simulink model "SVM"  (R2018b)
settings: Solver=VariableStepAuto  StartTime=0.0  StopTime=0.1  FixedStep=1/100000000  RelTol=1e-3
PostLoadFcn:
  | , if any(exist('dsrtsu_mdlpostloadfcn', 'file') ~= 0), dsrtsu_mdlpostloadfcn('Execute', bdroot); end,
values from neighbouring files (symbols this model uses):
  omega = 75    [param.m]
  Vo = 200    [param.m]
libraries: xbsIndex_r4 x2079, xrbsSSR_Library x20, xrbsMath_r4 x11, rtiproclib x6, rtifpgainterfacelib x1, powerlib_meascontrol x1
(part 4 of 23)

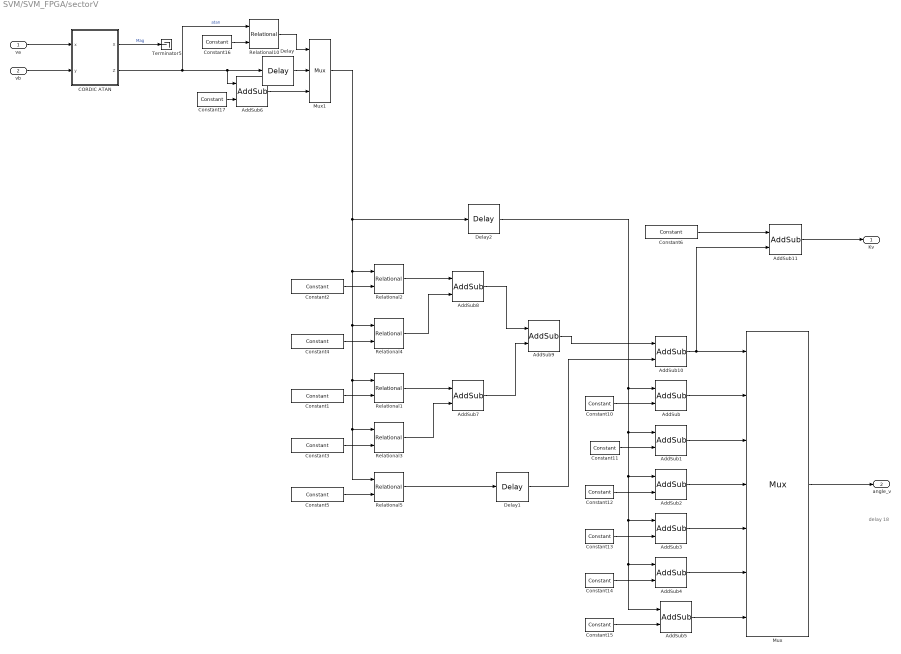
== system SVM/SVM_FPGA/sectorV ==
  note: delay 18
  va : Inport
  vb : Inport  Port=2
  AddSub{,1..5} (6 alike) : xbsIndex_r4/AddSub  mode=Subtraction  use_carryin=off  use_carryout=off  en=off  latency=1  precision=User Defined  arith_type="Signed  (2's comp)"  n_bits=16  bin_pt=8  quantization=Truncate  overflow=Wrap  use_behavioral_HDL=off  hw_selection=Fabric  pipelined=off  dbl_ovrd=off  block_type=addsub
  AddSub10 : xbsIndex_r4/AddSub  mode=Addition  use_carryin=off  use_carryout=off  en=off  latency=1  precision=User Defined  arith_type=Unsigned  n_bits=3  bin_pt=0  quantization=Truncate  overflow=Wrap  use_behavioral_HDL=off  hw_selection=Fabric  pipelined=off  dbl_ovrd=off  block_type=addsub
  AddSub11 : xbsIndex_r4/AddSub  mode=Addition  use_carryin=off  use_carryout=off  en=off  latency=1  precision=User Defined  arith_type=Unsigned  n_bits=3  bin_pt=0  quantization=Truncate  overflow=Wrap  use_behavioral_HDL=off  hw_selection=Fabric  pipelined=off  dbl_ovrd=off  block_type=addsub
  AddSub6 : xbsIndex_r4/AddSub  mode=Addition  use_carryin=off  use_carryout=off  en=off  latency=1  precision=User Defined  arith_type=Unsigned  n_bits=16  bin_pt=8  quantization=Truncate  overflow=Wrap  use_behavioral_HDL=off  hw_selection=Fabric  pipelined=off  dbl_ovrd=off  block_type=addsub
  AddSub7 : xbsIndex_r4/AddSub  mode=Addition  use_carryin=off  use_carryout=off  en=off  latency=1  precision=User Defined  arith_type=Unsigned  n_bits=2  bin_pt=0  quantization=Truncate  overflow=Wrap  use_behavioral_HDL=off  hw_selection=Fabric  pipelined=off  dbl_ovrd=off  block_type=addsub
  AddSub8 : xbsIndex_r4/AddSub  mode=Addition  use_carryin=off  use_carryout=off  en=off  latency=1  precision=User Defined  arith_type=Unsigned  n_bits=2  bin_pt=0  quantization=Truncate  overflow=Wrap  use_behavioral_HDL=off  hw_selection=Fabric  pipelined=off  dbl_ovrd=off  block_type=addsub
  AddSub9 : xbsIndex_r4/AddSub  mode=Addition  use_carryin=off  use_carryout=off  en=off  latency=1  precision=User Defined  arith_type=Unsigned  n_bits=3  bin_pt=0  quantization=Truncate  overflow=Wrap  use_behavioral_HDL=off  hw_selection=Fabric  pipelined=off  dbl_ovrd=off  block_type=addsub
  CORDIC ATAN : Subsystem  mask(Xilinx CORDIC ATAN){stages=25, pe_nbits=32, pe_binpt=8, pipeline_x=ones(1,8), prev_stages=25, pipeline=[1  1  1  1  1  1  1  1  0  0  0  0  0  0  0  0  0  0  0  0  0  0  0  0  0]}
      mask prompts: stages "Number of Processing Elements (integer value starting from 1)"; pe_nbits "X, Y Data Width"; pe_binpt "X, Y Binary Point Position"; pipeline_x "Latency for each Processing Element [1 0 0 1]"; prev_stages "Previous Number of Stages"; pipeline "Previous Pipeline Values"
      mask help: A parallel implementation, circular vectoring mode CORDIC processor for performing rectangular-to-polar conversion. The number of iteration stages (and resultant output accuracy) and the processor arithmetic precision are controlled by the mask customization.
      mask init:
      | [bg,fg] = xlcmap('XBlock',0);
      | iPos = get_param(gcb,'Position');
      | iWidth=iPos(3)-iPos(1); iHeight=iPos(4)-iPos(2);
      | iCx=iWidth/2;
      | iCy=iHeight/2;
      | [logoX, logoY] = xlogo(iPos);
      | sav_gcb=gcb;
      | stages = round(sum(abs(stages)));
      | if (stages == 0)
      | 	stages = prev_stages;
      | end
      | x = zeros(1,stages);
      | pipe_size = max(size(pipeline_x));
      | if pipe_size >= stages
      | 	x(1,1:stages) = pipeline_x(1,1:stages);
      | else
      | 	x(1,1:pipe_size) = pipeline_x(1,1:pipe_size);
      | end
      | 
      | if (stages ~=prev_stages)
      | 	pipeline=x;
      | 	cordic_pe = find_system(gcb, 'lookUnderMasks', 'all', 'FollowLinks','on','masktype', 'CORDIC parallel PE');
      |     
      |   a=find_system(cordic_pe{1}, 'lookUnderMasks', 'all', 'FollowLinks','on','masktype', 'CORDIC iteration PE');
      |   for i= 2:length(a)
      |     for j=1:3
      | 	  delete_line(cordic_pe{1}, ['CORDIC PE' int2str(i-1) '/' int2str(j)], ['CORDIC PE' int2str(i) '/' int2str(j)]);
      |     end
      |   end
      |     if length(a)>0,
      |       delete_line(cordic_pe{1}, 'x/1', 'CORDIC PE1/1');
      |       delete_line(cordic_pe{1}, 'y/1', 'CORDIC PE1/2');
      |       delete_line(cordic_pe{1}, 'z/1', 'CORDIC PE1/3');
      |       delete_line(cordic_pe{1}, ['CORDIC PE' int2str(length(a)) '/1'],'X/1');
      |       delete_line(cordic_pe{1}, ['CORDIC PE' int2str(length(a)) '/2'],'Terminator/1');
      |       delete_line(cordic_pe{1}, ['CORDIC PE' int2str(length(a)) '/3'],'Z/1');
      |     elseif length(a)==0
      |       temp_port=get_param([cordic_pe{1} '/x'],'porthandles');
      |       temp_line=get_param(temp_port.Outport,'line');
      |       if temp_line>=0  delete_line(temp_line); end
      |       temp_port=get_param([cordic_pe{1} '/y'],'porthandles');
      |       temp_line=get_param(temp_port.Outport,'line');
      |       if temp_line>=0  delete_line(temp_line); end
      |       temp_port=get_param([cordic_pe{1} '/z'],'porthandles');
      |       temp_line=get_param(temp_port.Outport,'line');
      |       if temp_line>=0  delete_line(temp_line); end
      |     end
      | 
      |     for i=2:length(a)
      |       delete_block(a{i});
      |     end
      |     for i=2:stages,
      |         add_block([cordic_pe{1} '/CORDIC PE1'], [cordic_pe{1} '/CORDIC PE' int2str(i)], 'ii', int2str(i-1),'pe_nbits', 'pe_nbits','pe_binpt', 'pe_binpt','pipeline',['pipeline(1,' int2str(i) ')'],'position',[150+(i-1)*125, 70, 205+(i-1)*125, 130]);
      |     end
      | 
      |     for i= 2:stages,
      |       for j=1:3
      | 		add_line(cordic_pe{1}, ['CORDIC PE' int2str(i-1) '/' int2str(j)], ['CORDIC PE' int2str(i) '/' int2str(j)], 'autorouting', 'on');
      |       end
      |     end
      | 
      |     if stages==0
      |       add_line(cordic_pe{1}, 'x/1', 'X/1', 'autorouting', 'on');
      |       add_line(cordic_pe{1}, 'y/1', 'Terminator/1', 'autorouting', 'on');
      |       add_line(cordic_pe{1}, 'z/1', 'Z/1', 'autorouting', 'on');
      |     elseif stages>0
      |       add_line(cordic_pe{1}, 'x/1', 'CORDIC PE1/1', 'autorouting', 'on');
      |       add_line(cordic_pe{1}, 'y/1', 'CORDIC PE1/2', 'autorouting', 'on');
      |       add_line(cordic_pe{1}, 'z/1', 'CORDIC PE1/3', 'autorouting', 'on');
      | 
      |       set_param([cordic_pe{1} '/' 'X'], 'Position', [150+stages*125, 72, 180+stages*125, 86]);
      |       set_param([cordic_pe{1} '/' 'Terminator'], 'Position', [210+stages*125, 92, 225+stages*125, 108]);
      |       set_param([cordic_pe{1} '/' 'Z'], 'Position', [240+stages*125, 113, 270+stages*125, 127]);
      | 
      |       add_line(cordic_pe{1}, ['CORDIC PE' int2str(stages) '/1'], 'X/1', 'autorouting', 'on');
      |       add_line(cordic_pe{1}, ['CORDIC PE' int2str(stages) '/2'], 'Terminator/1', 'autorouting', 'on');
      |       add_line(cordic_pe{1}, ['CORDIC PE' int2str(stages) '/3'],'Z/1', 'autorouting', 'on');
      | 
      |       % force a "compile" of the constituent constant blocks to
      |       % workaround a data propagation problem
      |       find_system(cordic_pe{1}, 'lookUnderMasks', 'all', 'FollowLinks', 'on', 'MaskType','Xilinx Constant Block');
      |   end
      | 	set_param(sav_gcb, 'prev_stages', int2str(stages));
      | 	set_param(sav_gcb, 'pipeline', [ '[' int2str(x) ']']);
      | else
      | 	if (sum(pipeline~=x))
      | 		set_param(gcb, 'pipeline', [ '[' int2str(x) ']']);
      | 	end
      | end
      | str = sprintf('-%d',sum(x) + 3);
      settings: CopyFcn=set_param(gcb, 'MaskSelfModifiable', 'on', 'LinkStatus', 'none');
      mask Help: eval('');xlDoc('-book','sysgen','-topic','CORDIC_ATAN');
      mask Display:
      | patch([0 iWidth iWidth 0],[0 0 iHeight iHeight] , bg);
      | patch(logoX,logoY , fg);
      | text(iCx-6,iCy,'z');
      | text(iCx,iCy+4,str);
      | port_label('input',1,'x');
      | port_label('input',2,'y');
      | port_label('output',1,'mag');
      | port_label('output',2,'atan');
      | plot([0 0 iWidth iWidth 0], [0 iHeight iHeight 0 0]);
  Constant1 : xbsIndex_r4/Constant  const=pi  gui_display_data_type=Fixed-point  arith_type=Signed (2's comp)  n_bits=16  bin_pt=8  preci_type=Single  exp_width=8  frac_width=24  explicit_period=off  period=1  equ=P=C  opselect=C  inp2=PCIN>>17  opr=+  inp1=P  carry=CIN  dbl_ovrd=off  block_type=constant
  Constant10 : xbsIndex_r4/Constant  const=pi/6  gui_display_data_type=Fixed-point  arith_type=Signed (2's comp)  n_bits=16  bin_pt=8  preci_type=Single  exp_width=8  frac_width=24  explicit_period=off  period=1  equ=P=C  opselect=C  inp2=PCIN>>17  opr=+  inp1=P  carry=CIN  dbl_ovrd=off  block_type=constant
  Constant11 : xbsIndex_r4/Constant  const=pi/2  gui_display_data_type=Fixed-point  arith_type=Signed (2's comp)  n_bits=16  bin_pt=8  preci_type=Single  exp_width=8  frac_width=24  explicit_period=off  period=1  equ=P=C  opselect=C  inp2=PCIN>>17  opr=+  inp1=P  carry=CIN  dbl_ovrd=off  block_type=constant
  Constant12 : xbsIndex_r4/Constant  const=5*pi/6  gui_display_data_type=Fixed-point  arith_type=Signed (2's comp)  n_bits=16  bin_pt=8  preci_type=Single  exp_width=8  frac_width=24  explicit_period=off  period=1  equ=P=C  opselect=C  inp2=PCIN>>17  opr=+  inp1=P  carry=CIN  dbl_ovrd=off  block_type=constant
  Constant13 : xbsIndex_r4/Constant  const=7*pi/6  gui_display_data_type=Fixed-point  arith_type=Signed (2's comp)  n_bits=16  bin_pt=8  preci_type=Single  exp_width=8  frac_width=24  explicit_period=off  period=1  equ=P=C  opselect=C  inp2=PCIN>>17  opr=+  inp1=P  carry=CIN  dbl_ovrd=off  block_type=constant
  Constant14 : xbsIndex_r4/Constant  const=3*pi/2  gui_display_data_type=Fixed-point  arith_type=Signed (2's comp)  n_bits=16  bin_pt=8  preci_type=Single  exp_width=8  frac_width=24  explicit_period=off  period=1  equ=P=C  opselect=C  inp2=PCIN>>17  opr=+  inp1=P  carry=CIN  dbl_ovrd=off  block_type=constant
  Constant15 : xbsIndex_r4/Constant  const=11*pi/6  gui_display_data_type=Fixed-point  arith_type=Signed (2's comp)  n_bits=16  bin_pt=8  preci_type=Single  exp_width=8  frac_width=24  explicit_period=off  period=1  equ=P=C  opselect=C  inp2=PCIN>>17  opr=+  inp1=P  carry=CIN  dbl_ovrd=off  block_type=constant
  Constant16 : xbsIndex_r4/Constant  const=0.0  gui_display_data_type=Fixed-point  arith_type=Signed (2's comp)  n_bits=16  bin_pt=8  preci_type=Single  exp_width=8  frac_width=24  explicit_period=off  period=1  equ=P=C  opselect=C  inp2=PCIN>>17  opr=+  inp1=P  carry=CIN  dbl_ovrd=off  block_type=constant
  Constant17 : xbsIndex_r4/Constant  const=2*pi  gui_display_data_type=Fixed-point  arith_type=Signed (2's comp)  n_bits=16  bin_pt=8  preci_type=Single  exp_width=8  frac_width=24  explicit_period=off  period=1  equ=P=C  opselect=C  inp2=PCIN>>17  opr=+  inp1=P  carry=CIN  dbl_ovrd=off  block_type=constant
  Constant2 : xbsIndex_r4/Constant  const=pi/3  gui_display_data_type=Fixed-point  arith_type=Signed (2's comp)  n_bits=16  bin_pt=8  preci_type=Single  exp_width=8  frac_width=24  explicit_period=off  period=1  equ=P=C  opselect=C  inp2=PCIN>>17  opr=+  inp1=P  carry=CIN  dbl_ovrd=off  block_type=constant
  Constant3 : xbsIndex_r4/Constant  const=4*pi/3  gui_display_data_type=Fixed-point  arith_type=Signed (2's comp)  n_bits=16  bin_pt=8  preci_type=Single  exp_width=8  frac_width=24  explicit_period=off  period=1  equ=P=C  opselect=C  inp2=PCIN>>17  opr=+  inp1=P  carry=CIN  dbl_ovrd=off  block_type=constant
  Constant4 : xbsIndex_r4/Constant  const=2*pi/3  gui_display_data_type=Fixed-point  arith_type=Signed (2's comp)  n_bits=16  bin_pt=8  preci_type=Single  exp_width=8  frac_width=24  explicit_period=off  period=1  equ=P=C  opselect=C  inp2=PCIN>>17  opr=+  inp1=P  carry=CIN  dbl_ovrd=off  block_type=constant
  Constant5 : xbsIndex_r4/Constant  const=5*pi/3  gui_display_data_type=Fixed-point  arith_type=Signed (2's comp)  n_bits=16  bin_pt=8  preci_type=Single  exp_width=8  frac_width=24  explicit_period=off  period=1  equ=P=C  opselect=C  inp2=PCIN>>17  opr=+  inp1=P  carry=CIN  dbl_ovrd=off  block_type=constant
  Constant6 : xbsIndex_r4/Constant  const=1  gui_display_data_type=Fixed-point  arith_type=Signed (2's comp)  n_bits=3  bin_pt=0  preci_type=Single  exp_width=8  frac_width=24  explicit_period=off  period=1  equ=P=C  opselect=C  inp2=PCIN>>17  opr=+  inp1=P  carry=CIN  dbl_ovrd=off  block_type=constant
  Delay : xbsIndex_r4/Delay  rst=off  infoeditControl=Selection of Reset will increase slice count due to use of real FFs and instead of SRLs  en=off  latency=1  reg_retiming=off  dbl_ovrd=off  block_type=delay
  Delay1 : xbsIndex_r4/Delay  rst=off  infoeditControl=Selection of Reset will increase slice count due to use of real FFs and instead of SRLs  en=off  latency=2  reg_retiming=off  dbl_ovrd=off  block_type=delay
  Delay2 : xbsIndex_r4/Delay  rst=off  infoeditControl=Selection of Reset will increase slice count due to use of real FFs and instead of SRLs  en=off  latency=3  reg_retiming=off  dbl_ovrd=off  block_type=delay
  Mux : xbsIndex_r4/Mux  inputs=6  en=off  latency=1  precision=User Defined  arith_type="Signed  (2's comp)"  n_bits=16  bin_pt=8  quantization=Truncate  overflow=Wrap  dbl_ovrd=off  block_type=mux
  Mux1 : xbsIndex_r4/Mux  inputs=2  en=off  latency=1  precision=User Defined  arith_type="Signed  (2's comp)"  n_bits=16  bin_pt=8  quantization=Truncate  overflow=Wrap  dbl_ovrd=off  block_type=mux
  Relational{1..5} (5 alike) : xbsIndex_r4/Relational  mode=a>=b  op_type=Ufix  en=off  latency=1  dbl_ovrd=off  block_type=relational
  Relational10 : xbsIndex_r4/Relational  mode=a<b  op_type=Bool  en=off  latency=1  dbl_ovrd=off  block_type=relational
  Terminator5 : Terminator
  Kv : Outport
  angle_v : Outport  Port=2
  wires:
  Constant14/1 -> AddSub4/2
  Constant12/1 -> AddSub2/2
  Constant10/1 -> AddSub/2
  Delay1/1 -> AddSub10/2
  Constant11/1 -> AddSub1/2
  Relational2/1 -> AddSub8/1
  Constant5/1 -> Relational5/2
  Delay2/1 -> AddSub4/1, AddSub5/1, AddSub3/1, AddSub2/1, AddSub1/1, AddSub/1
  va/1 -> CORDIC ATAN/1(x)
  Constant4/1 -> Relational4/2
  Mux1/1 -> Relational5/1, Relational3/1, Relational1/1, Relational4/1, Relational2/1, Delay2/1
  Constant16/1 -> Relational10/2
  CORDIC ATAN/1(X) -> Terminator5/1  "Mag"
  Constant17/1 -> AddSub6/2
  AddSub/1 -> Mux/2
  AddSub2/1 -> Mux/4
  AddSub5/1 -> Mux/7
  CORDIC ATAN/2(Z) -> Relational10/1, AddSub6/1, Delay/1  "atan"
  vb/1 -> CORDIC ATAN/2(y)
  Delay/1 -> Mux1/2
  Relational4/1 -> AddSub8/2
  Constant2/1 -> Relational2/2
  AddSub8/1 -> AddSub9/1
  AddSub1/1 -> Mux/3
  Relational1/1 -> AddSub7/1
  Constant3/1 -> Relational3/2
  Relational10/1 -> Mux1/1
  AddSub9/1 -> AddSub10/1
  AddSub11/1 -> Kv/1
  Constant1/1 -> Relational1/2
  AddSub4/1 -> Mux/6
  Relational3/1 -> AddSub7/2
  AddSub6/1 -> Mux1/3
  AddSub3/1 -> Mux/5
  AddSub7/1 -> AddSub9/2
  Constant6/1 -> AddSub11/1
  Relational5/1 -> Delay1/1
  Constant13/1 -> AddSub3/2
  AddSub10/1 -> AddSub11/2, Mux/1
  Constant15/1 -> AddSub5/2
  Mux/1 -> angle_v/1

== system SVM/SVM_FPGA/select_vector ==
  vector : Inport
  +1 : xbsIndex_r4/Constant  const=19  gui_display_data_type=Fixed-point  arith_type=Unsigned  n_bits=9  bin_pt=0  preci_type=Single  exp_width=8  frac_width=24  explicit_period=off  period=1  equ=P=C  opselect=C  inp2=PCIN>>17  opr=+  inp1=P  carry=CIN  dbl_ovrd=off  block_type=constant
  +{2..9} (8 alike) : xbsIndex_r4/Constant  const=19  gui_display_data_type=Fixed-point  arith_type=Signed (2's comp)  n_bits=16  bin_pt=8  preci_type=Single  exp_width=8  frac_width=24  explicit_period=off  period=1  equ=P=C  opselect=C  inp2=PCIN>>17  opr=+  inp1=P  carry=CIN  dbl_ovrd=off  block_type=constant
  -{1..9} (9 alike) : xbsIndex_r4/Constant  const=19  gui_display_data_type=Fixed-point  arith_type=Signed (2's comp)  n_bits=16  bin_pt=8  preci_type=Single  exp_width=8  frac_width=24  explicit_period=off  period=1  equ=P=C  opselect=C  inp2=PCIN>>17  opr=+  inp1=P  carry=CIN  dbl_ovrd=off  block_type=constant
  0a : xbsIndex_r4/Constant  const=19  gui_display_data_type=Fixed-point  arith_type=Signed (2's comp)  n_bits=16  bin_pt=8  preci_type=Single  exp_width=8  frac_width=24  explicit_period=off  period=1  equ=P=C  opselect=C  inp2=PCIN>>17  opr=+  inp1=P  carry=CIN  dbl_ovrd=off  block_type=constant
  0b : xbsIndex_r4/Constant  const=19  gui_display_data_type=Fixed-point  arith_type=Signed (2's comp)  n_bits=16  bin_pt=8  preci_type=Single  exp_width=8  frac_width=24  explicit_period=off  period=1  equ=P=C  opselect=C  inp2=PCIN>>17  opr=+  inp1=P  carry=CIN  dbl_ovrd=off  block_type=constant
  0c : xbsIndex_r4/Constant  const=19  gui_display_data_type=Fixed-point  arith_type=Signed (2's comp)  n_bits=16  bin_pt=8  preci_type=Single  exp_width=8  frac_width=24  explicit_period=off  period=1  equ=P=C  opselect=C  inp2=PCIN>>17  opr=+  inp1=P  carry=CIN  dbl_ovrd=off  block_type=constant
  Mux1 : xbsIndex_r4/Mux  inputs=21  en=off  latency=1  precision=Full  arith_type=Unsigned  n_bits=16  bin_pt=14  quantization=Truncate  overflow=Wrap  dbl_ovrd=off  block_type=mux
  switches : Outport
  wires:
  +3/1 -> Mux1/6
  +2/1 -> Mux1/4
  +1/1 -> Mux1/2
  +7/1 -> Mux1/14
  +8/1 -> Mux1/16
  -2/1 -> Mux1/5
  -3/1 -> Mux1/7
  -4/1 -> Mux1/9
  -7/1 -> Mux1/15
  +5/1 -> Mux1/10
  0c/1 -> Mux1/22
  0b/1 -> Mux1/21
  -8/1 -> Mux1/17
  +4/1 -> Mux1/8
  +9/1 -> Mux1/18
  +6/1 -> Mux1/12
  -5/1 -> Mux1/11
  vector/1 -> Mux1/1
  -6/1 -> Mux1/13
  -9/1 -> Mux1/19
  -1/1 -> Mux1/3
  0a/1 -> Mux1/20
  Mux1/1 -> switches/1

== system SVM/SVM_FPGA/ticks_calculator ==
  note: delay 6
  ticks_per_period : Inport
  d1 : Inport  Port=2
  d2 : Inport  Port=3
  d3 : Inport  Port=4
  d4 : Inport  Port=5
  AddSub : xbsIndex_r4/AddSub  mode=Addition  use_carryin=off  use_carryout=off  en=off  latency=1  precision=Full  arith_type=Unsigned  n_bits=16  bin_pt=14  quantization=Truncate  overflow=Wrap  use_behavioral_HDL=off  hw_selection=Fabric  pipelined=off  dbl_ovrd=off  block_type=addsub
  AddSub1 : xbsIndex_r4/AddSub  mode=Addition  use_carryin=off  use_carryout=off  en=off  latency=1  precision=Full  arith_type=Unsigned  n_bits=16  bin_pt=14  quantization=Truncate  overflow=Wrap  use_behavioral_HDL=off  hw_selection=Fabric  pipelined=off  dbl_ovrd=off  block_type=addsub
  AddSub2 : xbsIndex_r4/AddSub  mode=Subtraction  use_carryin=off  use_carryout=off  en=off  latency=1  precision=Full  arith_type=Unsigned  n_bits=16  bin_pt=14  quantization=Truncate  overflow=Wrap  use_behavioral_HDL=off  hw_selection=Fabric  pipelined=off  dbl_ovrd=off  block_type=addsub
  AddSub3 : xbsIndex_r4/AddSub  mode=Addition  use_carryin=off  use_carryout=off  en=off  latency=1  precision=Full  arith_type=Unsigned  n_bits=16  bin_pt=14  quantization=Truncate  overflow=Wrap  use_behavioral_HDL=off  hw_selection=Fabric  pipelined=off  dbl_ovrd=off  block_type=addsub
  Delay{,1..3} (4 alike) : xbsIndex_r4/Delay  rst=off  infoeditControl=Selection of Reset will increase slice count due to use of real FFs and instead of SRLs  en=off  latency=3  reg_retiming=off  dbl_ovrd=off  block_type=delay
  Mult{,1..3} (4 alike) : xbsIndex_r4/Mult  precision=Full  arith_type="Signed  (2's comp)"  n_bits=16  bin_pt=14  quantization=Truncate  overflow=Wrap  en=off  latency=3  use_behavioral_HDL=off  opt=Speed  use_embedded=on  optimum_pipeline=off  pipeline=on  dbl_ovrd=off  use_rpm=on  placement_style=Triangular  block_type=mult
  d0_counts : Outport
  d1_counts : Outport  Port=2
  d2_counts : Outport  Port=3
  d3_counts : Outport  Port=4
  "d4_counts " : Outport  Port=5
  wires:
  ticks_per_period/1 -> AddSub2/1, Mult1/2, Mult2/2, Mult3/2, Mult/2
  Mult/1 -> Delay/1, AddSub/1
  d1/1 -> Mult/1
  Mult2/1 -> AddSub1/1, Delay2/1
  d4/1 -> Mult3/1
  Mult3/1 -> Delay3/1, AddSub1/2
  AddSub1/1 -> AddSub3/2
  Mult1/1 -> Delay1/1, AddSub/2
  d2/1 -> Mult1/1
  AddSub/1 -> AddSub3/1
  AddSub3/1 -> AddSub2/2
  d3/1 -> Mult2/1
  AddSub2/1 -> d0_counts/1
  Delay/1 -> d1_counts/1
  Delay1/1 -> d2_counts/1
  Delay2/1 -> d3_counts/1
  Delay3/1 -> "d4_counts "/1

== system SVM/SVM_FPGA/vector_selector ==
  note: delay 1
  sector : Inport
  Demux : Demux
  Vector Constant : xrbsSSR_Library/Vector Constant  const=[17 14 6 1]  gui_display_data_type=Fixed-point  arith_type=Signed (2's comp)  n_bits=5  bin_pt=0  preci_type=Single  exp_width=8  frac_width=24  explicit_period=off  period=1  sg_ssr=4  sg_ssr_prev=4  equ=P=C  opselect=C  inp2=PCIN>>17  opr=+  inp1=P  carry=CIN  dbl_ovrd=off  block_type=constant_ssr
      settings: SourceProductName=Xilinx SSR Blockset
  Vector Constant1 : xrbsSSR_Library/Vector Constant  const=[16 17 3 6]  gui_display_data_type=Fixed-point  arith_type=Signed (2's comp)  n_bits=5  bin_pt=0  preci_type=Single  exp_width=8  frac_width=24  explicit_period=off  period=1  sg_ssr=4  sg_ssr_prev=4  equ=P=C  opselect=C  inp2=PCIN>>17  opr=+  inp1=P  carry=CIN  dbl_ovrd=off  block_type=constant_ssr
      settings: SourceProductName=Xilinx SSR Blockset
  Vector Constant10 : xrbsSSR_Library/Vector Constant  const=[15 18 4 5]  gui_display_data_type=Fixed-point  arith_type=Signed (2's comp)  n_bits=5  bin_pt=0  preci_type=Single  exp_width=8  frac_width=24  explicit_period=off  period=1  sg_ssr=4  sg_ssr_prev=4  equ=P=C  opselect=C  inp2=PCIN>>17  opr=+  inp1=P  carry=CIN  dbl_ovrd=off  block_type=constant_ssr
      settings: SourceProductName=Xilinx SSR Blockset
  Vector Constant11 : xrbsSSR_Library/Vector Constant  const=[14 15 1 4]  gui_display_data_type=Fixed-point  arith_type=Signed (2's comp)  n_bits=5  bin_pt=0  preci_type=Single  exp_width=8  frac_width=24  explicit_period=off  period=1  sg_ssr=4  sg_ssr_prev=4  equ=P=C  opselect=C  inp2=PCIN>>17  opr=+  inp1=P  carry=CIN  dbl_ovrd=off  block_type=constant_ssr
      settings: SourceProductName=Xilinx SSR Blockset
  Vector Constant12 : xrbsSSR_Library/Vector Constant  const=[11 8 18 13]  gui_display_data_type=Fixed-point  arith_type=Signed (2's comp)  n_bits=5  bin_pt=0  preci_type=Single  exp_width=8  frac_width=24  explicit_period=off  period=1  sg_ssr=4  sg_ssr_prev=4  equ=P=C  opselect=C  inp2=PCIN>>17  opr=+  inp1=P  carry=CIN  dbl_ovrd=off  block_type=constant_ssr
      settings: SourceProductName=Xilinx SSR Blockset
  Vector Constant13 : xrbsSSR_Library/Vector Constant  const=[10 11 15 18]  gui_display_data_type=Fixed-point  arith_type=Signed (2's comp)  n_bits=5  bin_pt=0  preci_type=Single  exp_width=8  frac_width=24  explicit_period=off  period=1  sg_ssr=4  sg_ssr_prev=4  equ=P=C  opselect=C  inp2=PCIN>>17  opr=+  inp1=P  carry=CIN  dbl_ovrd=off  block_type=constant_ssr
      settings: SourceProductName=Xilinx SSR Blockset
  Vector Constant14 : xrbsSSR_Library/Vector Constant  const=[7 10 14 15]  gui_display_data_type=Fixed-point  arith_type=Signed (2's comp)  n_bits=5  bin_pt=0  preci_type=Single  exp_width=8  frac_width=24  explicit_period=off  period=1  sg_ssr=4  sg_ssr_prev=4  equ=P=C  opselect=C  inp2=PCIN>>17  opr=+  inp1=P  carry=CIN  dbl_ovrd=off  block_type=constant_ssr
      settings: SourceProductName=Xilinx SSR Blockset
  Vector Constant15 : xrbsSSR_Library/Vector Constant  const=[6 1 11 8]  gui_display_data_type=Fixed-point  arith_type=Signed (2's comp)  n_bits=5  bin_pt=0  preci_type=Single  exp_width=8  frac_width=24  explicit_period=off  period=1  sg_ssr=4  sg_ssr_prev=4  equ=P=C  opselect=C  inp2=PCIN>>17  opr=+  inp1=P  carry=CIN  dbl_ovrd=off  block_type=constant_ssr
      settings: SourceProductName=Xilinx SSR Blockset
  Vector Constant16 : xrbsSSR_Library/Vector Constant  const=[3 6 10 11]  gui_display_data_type=Fixed-point  arith_type=Signed (2's comp)  n_bits=5  bin_pt=0  preci_type=Single  exp_width=8  frac_width=24  explicit_period=off  period=1  sg_ssr=4  sg_ssr_prev=4  equ=P=C  opselect=C  inp2=PCIN>>17  opr=+  inp1=P  carry=CIN  dbl_ovrd=off  block_type=constant_ssr
      settings: SourceProductName=Xilinx SSR Blockset
  Vector Constant17 : xrbsSSR_Library/Vector Constant  const=[2 3 7 10]  gui_display_data_type=Fixed-point  arith_type=Signed (2's comp)  n_bits=5  bin_pt=0  preci_type=Single  exp_width=8  frac_width=24  explicit_period=off  period=1  sg_ssr=4  sg_ssr_prev=4  equ=P=C  opselect=C  inp2=PCIN>>17  opr=+  inp1=P  carry=CIN  dbl_ovrd=off  block_type=constant_ssr
      settings: SourceProductName=Xilinx SSR Blockset
  Vector Constant18 : xrbsSSR_Library/Vector Constant  const=[19 19 19 19]  gui_display_data_type=Fixed-point  arith_type=Signed (2's comp)  n_bits=5  bin_pt=0  preci_type=Single  exp_width=8  frac_width=24  explicit_period=off  period=1  sg_ssr=4  sg_ssr_prev=4  equ=P=C  opselect=C  inp2=PCIN>>17  opr=+  inp1=P  carry=CIN  dbl_ovrd=off  block_type=constant_ssr
      settings: SourceProductName=Xilinx SSR Blockset
  Vector Constant2 : xrbsSSR_Library/Vector Constant  const=[13 16 2 3]  gui_display_data_type=Fixed-point  arith_type=Signed (2's comp)  n_bits=5  bin_pt=0  preci_type=Single  exp_width=8  frac_width=24  explicit_period=off  period=1  sg_ssr=4  sg_ssr_prev=4  equ=P=C  opselect=C  inp2=PCIN>>17  opr=+  inp1=P  carry=CIN  dbl_ovrd=off  block_type=constant_ssr
      settings: SourceProductName=Xilinx SSR Blockset
  Vector Constant3 : xrbsSSR_Library/Vector Constant  const=[12 7 17 14]  gui_display_data_type=Fixed-point  arith_type=Signed (2's comp)  n_bits=5  bin_pt=0  preci_type=Single  exp_width=8  frac_width=24  explicit_period=off  period=1  sg_ssr=4  sg_ssr_prev=4  equ=P=C  opselect=C  inp2=PCIN>>17  opr=+  inp1=P  carry=CIN  dbl_ovrd=off  block_type=constant_ssr
      settings: SourceProductName=Xilinx SSR Blockset
  Vector Constant4 : xrbsSSR_Library/Vector Constant  const=[9 12 16 17]  gui_display_data_type=Fixed-point  arith_type=Signed (2's comp)  n_bits=5  bin_pt=0  preci_type=Single  exp_width=8  frac_width=24  explicit_period=off  period=1  sg_ssr=4  sg_ssr_prev=4  equ=P=C  opselect=C  inp2=PCIN>>17  opr=+  inp1=P  carry=CIN  dbl_ovrd=off  block_type=constant_ssr
      settings: SourceProductName=Xilinx SSR Blockset
  Vector Constant5 : xrbsSSR_Library/Vector Constant  const=[8 9 13 16]  gui_display_data_type=Fixed-point  arith_type=Signed (2's comp)  n_bits=5  bin_pt=0  preci_type=Single  exp_width=8  frac_width=24  explicit_period=off  period=1  sg_ssr=4  sg_ssr_prev=4  equ=P=C  opselect=C  inp2=PCIN>>17  opr=+  inp1=P  carry=CIN  dbl_ovrd=off  block_type=constant_ssr
      settings: SourceProductName=Xilinx SSR Blockset
  Vector Constant6 : xrbsSSR_Library/Vector Constant  const=[5 2 12 7]  gui_display_data_type=Fixed-point  arith_type=Signed (2's comp)  n_bits=5  bin_pt=0  preci_type=Single  exp_width=8  frac_width=24  explicit_period=off  period=1  sg_ssr=4  sg_ssr_prev=4  equ=P=C  opselect=C  inp2=PCIN>>17  opr=+  inp1=P  carry=CIN  dbl_ovrd=off  block_type=constant_ssr
      settings: SourceProductName=Xilinx SSR Blockset
  Vector Constant7 : xrbsSSR_Library/Vector Constant  const=[4 5 9 12]  gui_display_data_type=Fixed-point  arith_type=Signed (2's comp)  n_bits=5  bin_pt=0  preci_type=Single  exp_width=8  frac_width=24  explicit_period=off  period=1  sg_ssr=4  sg_ssr_prev=4  equ=P=C  opselect=C  inp2=PCIN>>17  opr=+  inp1=P  carry=CIN  dbl_ovrd=off  block_type=constant_ssr
      settings: SourceProductName=Xilinx SSR Blockset
  Vector Constant8 : xrbsSSR_Library/Vector Constant  const=[1 4 8 9]  gui_display_data_type=Fixed-point  arith_type=Signed (2's comp)  n_bits=5  bin_pt=0  preci_type=Single  exp_width=8  frac_width=24  explicit_period=off  period=1  sg_ssr=4  sg_ssr_prev=4  equ=P=C  opselect=C  inp2=PCIN>>17  opr=+  inp1=P  carry=CIN  dbl_ovrd=off  block_type=constant_ssr
      settings: SourceProductName=Xilinx SSR Blockset
  Vector Constant9 : xrbsSSR_Library/Vector Constant  const=[18 13 5 2]  gui_display_data_type=Fixed-point  arith_type=Signed (2's comp)  n_bits=5  bin_pt=0  preci_type=Single  exp_width=8  frac_width=24  explicit_period=off  period=1  sg_ssr=4  sg_ssr_prev=4  equ=P=C  opselect=C  inp2=PCIN>>17  opr=+  inp1=P  carry=CIN  dbl_ovrd=off  block_type=constant_ssr
      settings: SourceProductName=Xilinx SSR Blockset
  Vector Mux : xrbsSSR_Library/Vector Mux  inputs=32  inputs_prev=31  en=off  vectorize_en=off  vectorize_sel=off  sg_latency=1  precision=User Defined  arith_type=Unsigned  n_bits=16  bin_pt=0  quantization=Truncate  overflow=Wrap  dbl_ovrd=off  block_type=mux_ssr  sg_ssr=4  sg_ssr_prev=4  sg_ssr_name=vect_mux
      settings: SourceProductName=Xilinx SSR Blockset  infoedit=The Vector Multiplexer block supports Multiplexing feature for input of vector types.
  "v1 " : Outport
  v2 : Outport  Port=2
  v3 : Outport  Port=3
  "v4 " : Outport  Port=4
  wires:
  Vector Mux/1 -> Demux/1
  Vector Constant/1 -> Vector Mux/2
  Vector Constant1/1 -> Vector Mux/3
  Vector Constant3/1 -> Vector Mux/5
  sector/1 -> Vector Mux/1
  Demux/1 -> "v1 "/1
  Demux/2 -> v2/1
  Demux/3 -> v3/1
  Demux/4 -> "v4 "/1
  Vector Constant2/1 -> Vector Mux/4
  Vector Constant4/1 -> Vector Mux/6
  Vector Constant5/1 -> Vector Mux/7
  Vector Constant6/1 -> Vector Mux/8
  Vector Constant7/1 -> Vector Mux/9
  Vector Constant8/1 -> Vector Mux/10
  Vector Constant9/1 -> Vector Mux/11
  Vector Constant10/1 -> Vector Mux/12
  Vector Constant11/1 -> Vector Mux/13
  Vector Constant12/1 -> Vector Mux/14
  Vector Constant13/1 -> Vector Mux/15
  Vector Constant14/1 -> Vector Mux/16
  Vector Constant15/1 -> Vector Mux/17
  Vector Constant16/1 -> Vector Mux/18
  Vector Constant17/1 -> Vector Mux/19
  Vector Constant18/1 -> Vector Mux/20, Vector Mux/21, Vector Mux/22, Vector Mux/23, Vector Mux/24, Vector Mux/25, Vector Mux/26, Vector Mux/27, Vector Mux/28, Vector Mux/29, Vector Mux/30, Vector Mux/31, Vector Mux/32, Vector Mux/33

== system SVM/SVM_FPGA/FPGA_XDATA_READ_BL1/phs_read_register ==
  note: Subsystem simulating the phs bus
      | access via RTLib functions.
  note: Subsystem simulating the communication
      | function specific behaviour. This is how the
      | FPGA framework driver takes effect on the data.
  data_i : Inport
  com_fct_model : Subsystem
  phs/rtlib_sim_model : Subsystem
  data_o : Outport
  data_new_o : Outport  Port=2
  wires:
  com_fct_model/2(data_new_o) -> data_new_o/1
  phs/rtlib_sim_model/1(data_o1) -> com_fct_model/1(data_i1)
  com_fct_model/1(data_o1) -> data_o/1
  data_i/1 -> phs/rtlib_sim_model/1(data_i1)

== system SVM/SVM_FPGA/FPGA_XDATA_READ_BL2/phs_read_register ==
  note: Subsystem simulating the phs bus
      | access via RTLib functions.
  note: Subsystem simulating the communication
      | function specific behaviour. This is how the
      | FPGA framework driver takes effect on the data.
  data_i : Inport
  com_fct_model : Subsystem
  phs/rtlib_sim_model : Subsystem
  data_o : Outport
  data_new_o : Outport  Port=2
  wires:
  com_fct_model/2(data_new_o) -> data_new_o/1
  phs/rtlib_sim_model/1(data_o1) -> com_fct_model/1(data_i1)
  com_fct_model/1(data_o1) -> data_o/1
  data_i/1 -> phs/rtlib_sim_model/1(data_i1)

== system SVM/SVM_FPGA/FPGA_XDATA_READ_BL3/phs_read_register ==
  note: Subsystem simulating the phs bus
      | access via RTLib functions.
  note: Subsystem simulating the communication
      | function specific behaviour. This is how the
      | FPGA framework driver takes effect on the data.
  data_i : Inport
  com_fct_model : Subsystem
  phs/rtlib_sim_model : Subsystem
  data_o : Outport
  data_new_o : Outport  Port=2
  wires:
  com_fct_model/2(data_new_o) -> data_new_o/1
  phs/rtlib_sim_model/1(data_o1) -> com_fct_model/1(data_i1)
  com_fct_model/1(data_o1) -> data_o/1
  data_i/1 -> phs/rtlib_sim_model/1(data_i1)

== system SVM/SVM_FPGA/FPGA_XDATA_READ_BL4/phs_read_register ==
  note: Subsystem simulating the phs bus
      | access via RTLib functions.
  note: Subsystem simulating the communication
      | function specific behaviour. This is how the
      | FPGA framework driver takes effect on the data.
  data_i : Inport
  com_fct_model : Subsystem
  phs/rtlib_sim_model : Subsystem
  data_o : Outport
  data_new_o : Outport  Port=2
  wires:
  com_fct_model/2(data_new_o) -> data_new_o/1
  phs/rtlib_sim_model/1(data_o1) -> com_fct_model/1(data_i1)
  com_fct_model/1(data_o1) -> data_o/1
  data_i/1 -> phs/rtlib_sim_model/1(data_i1)

== system SVM/SVM_FPGA/FPGA_XDATA_READ_BL5/phs_read_register ==
  note: Subsystem simulating the phs bus
      | access via RTLib functions.
  note: Subsystem simulating the communication
      | function specific behaviour. This is how the
      | FPGA framework driver takes effect on the data.
  data_i : Inport
  com_fct_model : Subsystem
  phs/rtlib_sim_model : Subsystem
  data_o : Outport
  data_new_o : Outport  Port=2
  wires:
  com_fct_model/2(data_new_o) -> data_new_o/1
  phs/rtlib_sim_model/1(data_o1) -> com_fct_model/1(data_i1)
  com_fct_model/1(data_o1) -> data_o/1
  data_i/1 -> phs/rtlib_sim_model/1(data_i1)

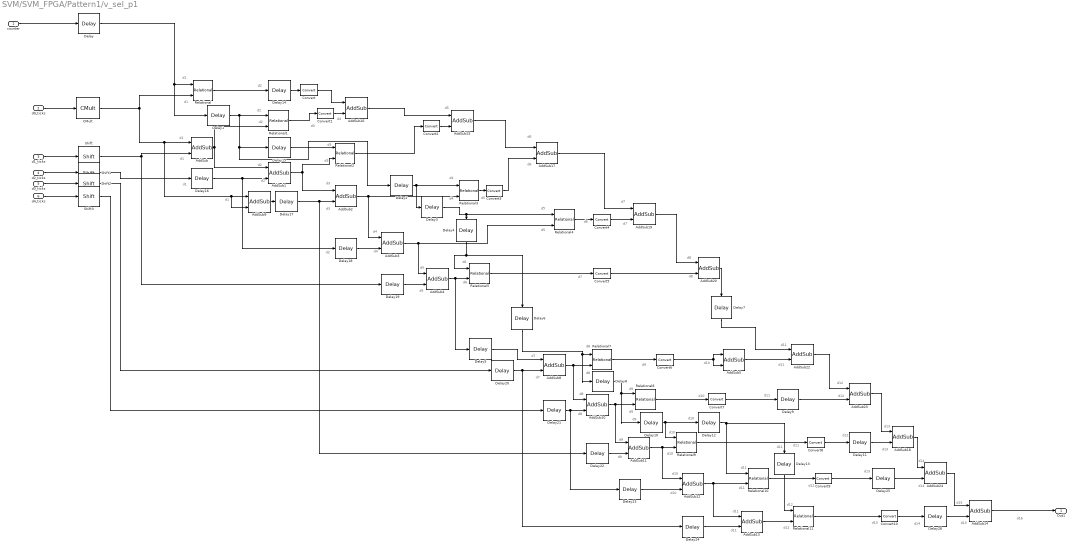
== system SVM/SVM_FPGA/Pattern1/v_sel_p1 ==
  note: d16
  note: d15
  note: d14
  note: d15
  note: d14
  note: d13
  note: d12
  note: d13
  note: d12
  note: d11
  note: d12
  note: d11
  note: d11
  note: d11
  note: d10
  note: d9
  note: d11
  note: d10
  note: d10
  note: d14
  note: d12
  note: d13
  note: d11
  note: d10
  note: d10
  note: d9
  note: d9
  note: d13
  note: d12
  note: d11
  note: d12
  note: d10
  note: d9
  note: d9
  note: d8
  note: d8
  note: d8
  note: d8
  note: d9
  note: d10
  note: d11
  note: d7
  note: d7
  note: d11
  note: d8
  note: d7
  note: d6
  note: d6
  note: d5
  note: d5
  note: d8
  note: d7
  note: d6
  note: d5
  note: d5
  note: d4
  note: d4
  note: d6
  note: d5
  note: d4
  note: d3
  note: d3
  note: d4
  note: d3
  note: d2
  note: d2
  note: d3
  note: d2
  note: d2
  note: d3
  note: d4
  note: d2
  note: d1
  note: d1
  note: d1
  note: d1
  note: d2
  note: d1
  note: d1
  note: d7
  note: d6
  note: d5
  counter : Inport
  d0_ticks : Inport  Port=2
  d1_ticks : Inport  Port=3
  d2_ticks : Inport  Port=4
  d3_ticks : Inport  Port=5
  d4_ticks : Inport  Port=6
  AddSub{,1..5,8..13,16} (13 alike) : xbsIndex_r4/AddSub  mode=Addition  use_carryin=off  use_carryout=off  en=off  latency=1  precision=Full  arith_type=Unsigned  n_bits=16  bin_pt=14  quantization=Truncate  overflow=Wrap  use_behavioral_HDL=off  hw_selection=Fabric  pipelined=off  dbl_ovrd=off  block_type=addsub
  AddSub{14,18,23..24} (4 alike) : xbsIndex_r4/AddSub  mode=Addition  use_carryin=off  use_carryout=off  en=off  latency=1  precision=User Defined  arith_type=Unsigned  n_bits=4  bin_pt=0  quantization=Truncate  overflow=Wrap  use_behavioral_HDL=off  hw_selection=Fabric  pipelined=off  dbl_ovrd=off  block_type=addsub
  AddSub15 : xbsIndex_r4/AddSub  mode=Addition  use_carryin=off  use_carryout=off  en=off  latency=1  precision=User Defined  arith_type=Unsigned  n_bits=2  bin_pt=0  quantization=Truncate  overflow=Wrap  use_behavioral_HDL=off  hw_selection=Fabric  pipelined=off  dbl_ovrd=off  block_type=addsub
  AddSub17 : xbsIndex_r4/AddSub  mode=Addition  use_carryin=off  use_carryout=off  en=off  latency=1  precision=User Defined  arith_type=Unsigned  n_bits=3  bin_pt=0  quantization=Truncate  overflow=Wrap  use_behavioral_HDL=off  hw_selection=Fabric  pipelined=off  dbl_ovrd=off  block_type=addsub
  AddSub19 : xbsIndex_r4/AddSub  mode=Addition  use_carryin=off  use_carryout=off  en=off  latency=1  precision=User Defined  arith_type=Unsigned  n_bits=3  bin_pt=0  quantization=Truncate  overflow=Wrap  use_behavioral_HDL=off  hw_selection=Fabric  pipelined=off  dbl_ovrd=off  block_type=addsub
  AddSub20 : xbsIndex_r4/AddSub  mode=Addition  use_carryin=off  use_carryout=off  en=off  latency=1  precision=User Defined  arith_type=Unsigned  n_bits=5  bin_pt=0  quantization=Truncate  overflow=Wrap  use_behavioral_HDL=off  hw_selection=Fabric  pipelined=off  dbl_ovrd=off  block_type=addsub
  AddSub22 : xbsIndex_r4/AddSub  mode=Addition  use_carryin=off  use_carryout=off  en=off  latency=1  precision=User Defined  arith_type=Unsigned  n_bits=3  bin_pt=0  quantization=Truncate  overflow=Wrap  use_behavioral_HDL=off  hw_selection=Fabric  pipelined=off  dbl_ovrd=off  block_type=addsub
  CMult : xbsIndex_r4/CMult  const=1/6  gui_display_data_type=Fixed-point  const_n_bits=16  const_bin_pt=16  float_type=Single  exp_bits=8  fraction_bits=24  en=off  latency=1  precision=Full  arith_type="Signed  (2's comp)"  n_bits=16  bin_pt=14  quantization=Truncate  overflow=Wrap  use_behavioral_HDL=off  mem_type=Distributed RAM  pipeline=off  dbl_ovrd=off  block_type=cmult
  Convert{,1..10} (11 alike) : xbsIndex_r4/Convert  gui_display_data_type=Fixed-point  arith_type="Signed  (2's comp)"  n_bits=1  bin_pt=0  float_type=Single  exp_bits=8  fraction_bits=24  quantization=Truncate  overflow=Wrap  en=off  latency=1  pipeline=off  dbl_ovrd=off  block_type=convert
  Delay{,1,3..5,8..17,25..26} (17 alike) : xbsIndex_r4/Delay  rst=off  infoeditControl=Selection of Reset will increase slice count due to use of real FFs and instead of SRLs  en=off  latency=1  reg_retiming=off  dbl_ovrd=off  block_type=delay
  Delay{2,6..7,18,23} (5 alike) : xbsIndex_r4/Delay  rst=off  infoeditControl=Selection of Reset will increase slice count due to use of real FFs and instead of SRLs  en=off  latency=2  reg_retiming=off  dbl_ovrd=off  block_type=delay
  Delay19 : xbsIndex_r4/Delay  rst=off  infoeditControl=Selection of Reset will increase slice count due to use of real FFs and instead of SRLs  en=off  latency=4  reg_retiming=off  dbl_ovrd=off  block_type=delay
  Delay20 : xbsIndex_r4/Delay  rst=off  infoeditControl=Selection of Reset will increase slice count due to use of real FFs and instead of SRLs  en=off  latency=6  reg_retiming=off  dbl_ovrd=off  block_type=delay
  Delay21 : xbsIndex_r4/Delay  rst=off  infoeditControl=Selection of Reset will increase slice count due to use of real FFs and instead of SRLs  en=off  latency=7  reg_retiming=off  dbl_ovrd=off  block_type=delay
  Delay22 : xbsIndex_r4/Delay  rst=off  infoeditControl=Selection of Reset will increase slice count due to use of real FFs and instead of SRLs  en=off  latency=6  reg_retiming=off  dbl_ovrd=off  block_type=delay
  Delay24 : xbsIndex_r4/Delay  rst=off  infoeditControl=Selection of Reset will increase slice count due to use of real FFs and instead of SRLs  en=off  latency=4  reg_retiming=off  dbl_ovrd=off  block_type=delay
  Relational{,1..5,7..11} (11 alike) : xbsIndex_r4/Relational  mode=a>b  op_type=Bool  en=off  latency=1  dbl_ovrd=off  block_type=relational
  Shift{,1..3} (4 alike) : xbsIndex_r4/Shift  shift_dir=Right  shift_bits=1  en=off  latency=1  precision=Full  arith_type="Signed  (2's comp)"  n_bits=16  bin_pt=14  quantization=Truncate  overflow=Wrap  dbl_ovrd=off  block_type=shift
  Out1 : Outport
  wires:
  AddSub15/1 -> AddSub17/1
  AddSub24/1 -> AddSub14/1
  Shift1/1 -> Delay16/1
  Delay17/1 -> AddSub2/2, Delay22/1
  AddSub11/1 -> AddSub12/1, Relational9/2
  Relational4/1 -> Convert4/1
  Delay19/1 -> AddSub4/2
  counter/1 -> Delay/1
  AddSub18/1 -> AddSub24/1
  CMult/1 -> Relational/2, AddSub9/2, AddSub9/1, AddSub/1
  Shift/1 -> Delay19/1, AddSub/2
  Delay20/1 -> Delay24/1, AddSub8/2
  Delay22/1 -> AddSub11/2
  Delay16/1 -> Delay18/1, AddSub1/2
  Relational1/1 -> Convert1/1
  AddSub12/1 -> AddSub13/1, Relational10/2
  Relational8/1 -> Convert7/1
  AddSub23/1 -> AddSub18/1
  Delay23/1 -> AddSub12/2
  Relational5/1 -> Convert5/1
  AddSub4/1 -> Delay5/1, Relational5/2
  AddSub/1 -> AddSub1/1, Relational1/2
  AddSub8/1 -> AddSub10/1, Relational7/2
  Delay15/1 -> Relational2/1
  Relational2/1 -> Convert2/1
  Delay14/1 -> Convert/1
  Delay21/1 -> Delay23/1, AddSub10/2
  d3_ticks/1 -> Shift2/1
  Relational10/1 -> Convert9/1
  AddSub19/1 -> AddSub20/1
  Delay18/1 -> AddSub3/2
  AddSub17/1 -> AddSub19/1
  Relational/1 -> Delay14/1
  AddSub1/1 -> AddSub2/1, Relational2/2
  AddSub22/1 -> AddSub23/1
  AddSub3/1 -> AddSub4/1, Relational4/2
  AddSub10/1 -> AddSub11/1, Relational8/2
  d1_ticks/1 -> Shift/1
  AddSub13/1 -> Relational11/2
  Delay24/1 -> AddSub13/2
  Shift2/1 -> Delay20/1
  Relational3/1 -> Convert3/1
  Relational11/1 -> Convert10/1
  AddSub2/1 -> AddSub3/1, Relational3/2
  AddSub20/1 -> Delay7/1
  Shift3/1 -> Delay21/1
  Relational7/1 -> Convert6/1
  Relational9/1 -> Convert8/1
  AddSub14/1 -> Out1/1
  d4_ticks/1 -> Shift3/1
  d2_ticks/1 -> Shift1/1
  AddSub9/1 -> Delay17/1
  AddSub5/1 -> AddSub22/2
  d0_ticks/1 -> CMult/1
  Convert/1 -> AddSub16/1
  Convert1/1 -> AddSub16/2
  AddSub16/1 -> AddSub15/1
  Convert2/1 -> AddSub15/2
  Convert3/1 -> AddSub17/2
  Convert4/1 -> AddSub19/2
  Convert5/1 -> AddSub20/2
  Convert6/1 -> AddSub5/1, AddSub5/2
  Convert7/1 -> Delay9/1
  Convert8/1 -> Delay11/1
  Convert9/1 -> Delay25/1
  Convert10/1 -> Delay26/1
  Delay/1 -> Delay1/1, Relational/1
  Delay1/1 -> Relational1/1, Delay15/1, Delay2/1
  Delay2/1 -> Relational3/1, Delay3/1
  Delay3/1 -> Relational4/1, Delay4/1
  Delay4/1 -> Delay6/1, Relational5/1
  Delay5/1 -> AddSub8/1
  Delay6/1 -> Delay8/1, Relational7/1
  Delay7/1 -> AddSub22/1
  Delay8/1 -> Delay10/1, Relational8/1
  Delay9/1 -> AddSub23/2
  Delay10/1 -> Relational9/1, Delay12/1
  Delay11/1 -> AddSub18/2
  Delay12/1 -> Delay13/1, Relational10/1
  Delay13/1 -> Relational11/1
  Delay25/1 -> AddSub24/2
  Delay26/1 -> AddSub14/2
